simulink model "nonlinear_observer"  (R2022a)
settings: Solver=VariableStepAuto  StartTime=0.0  StopTime=8  RelTol=1e-3
settings Model: SimulationMode=accelerator  Creator=dbagn  LastModifiedBy=dbagn

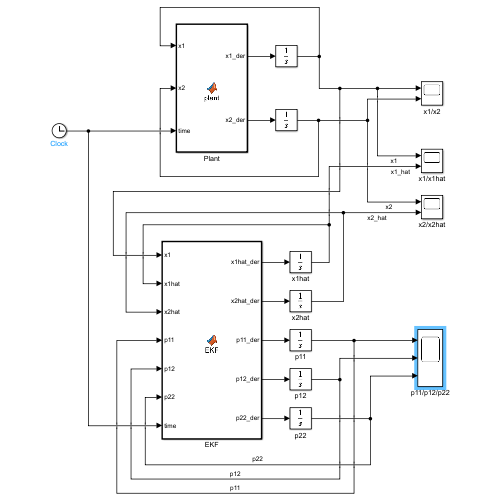
[thumbnail: Simulink's stored preview of the top-level diagram]
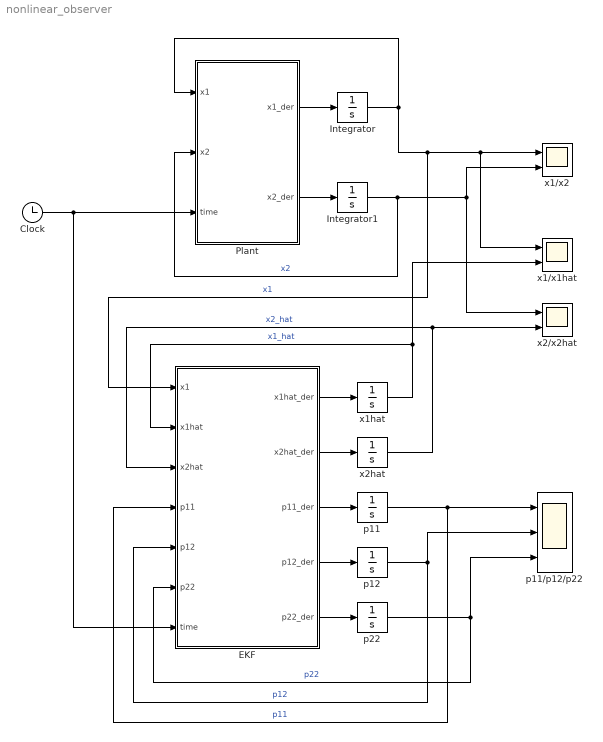
== system nonlinear_observer ==
  Clock : Clock
  EKF : MATLAB Function  TreatAsAtomicUnit=on
  Integrator : Integrator
  Integrator1 : Integrator
  Plant : MATLAB Function  TreatAsAtomicUnit=on
  p11 : Integrator
  p11/p12/p22 : Scope  NumInputPorts=3
  p12 : Integrator
  p22 : Integrator
  x1/x1hat : Scope  NumInputPorts=2
  x1/x2 : Scope  NumInputPorts=2
  x1hat : Integrator  InitialCondition=1
  x2/x2hat : Scope  NumInputPorts=2
  x2hat : Integrator  InitialCondition=-1
  wires:
  Clock/1 -> EKF/7(time), Plant/3(time)
  Integrator/1 -> EKF/1(x1), x1/x2/1, x1/x1hat/1, Plant/1(x1)  "x1"
  Plant/1(x1_der) -> Integrator/1
  Plant/2(x2_der) -> Integrator1/1
  Integrator1/1 -> Plant/2(x2), x1/x2/2, x2/x2hat/1  "x2"
  EKF/1(x1hat_der) -> x1hat/1
  EKF/2(x2hat_der) -> x2hat/1
  EKF/3(p11_der) -> p11/1
  EKF/4(p12_der) -> p12/1
  EKF/5(p22_der) -> p22/1
  x1hat/1 -> x1/x1hat/2, EKF/2(x1hat)  "x1_hat"
  x2hat/1 -> EKF/3(x2hat), x2/x2hat/2  "x2_hat"
  p11/1 -> EKF/4(p11), p11/p12/p22/1  "p11"
  p12/1 -> p11/p12/p22/2, EKF/5(p12)  "p12"
  p22/1 -> p11/p12/p22/3, EKF/6(p22)  "p22"

== matlab function nonlinear_observer/EKF ==
  data: x1 input; x1hat input; x1hat_der output; x2hat input; p11 input; p12 input; p22 input; time input; x2hat_der output; p11_der output; p12_der output; p22_der output
function [x1hat_der, x2hat_der, p11_der, p12_der, p22_der] = ...
    EKF(x1, x1hat, x2hat, p11, p12, p22, time)

x1hat_der = x2hat + p11*(x1-x1hat);
x2hat_der = -x1hat - 2*x2hat + (0.25*x1hat^2*x2hat + 0.2*sin(2*time)) + ...
    p12*(x1-x1hat);
p11_der = 2*p12+1-p11^2;
p12_der = p11*(-1+0.5*x1hat*x2hat)+p12*(-2+0.25*x1hat^2)+p22-p11*p12;
p22_der = 2*p12*(-1+0.5*x1hat*x2hat)+2*p22*(-2+0.25*x1hat^2)+1-p12^2;

== matlab function nonlinear_observer/Plant ==
  data: x1 input; x1_der output; x2 input; time input; x2_der output
function [x1_der, x2_der] = plant(x1, x2, time)
x1_der = x2;
x2_der = -x1-2*x2+(0.25*x1^2*x2+0.2*sin(2*time));
